simulink model "psk_rc_model"  (Simulink 8.7)
settings: Solver=FixedStepDiscrete  SolverMode=SingleTasking  StartTime=0.0  StopTime=1  FixedStep=1/100000  RelTol=1e-3  AbsTol=1e-6
undefined symbols (not defined in the file or in its folder): gcbh, rcfiltgaincompat
libraries: commfilt2 x1, dspsrcs4 x1
settings Model: Creator=amoura  LastModifiedBy=Artur Moura
settings DataIOCC: LimitDataPoints=off  SignalLoggingSaveFormat=ModelDataLogs
settings OptimizationCC: BlockReduction=off  BooleanDataType=off  ExpressionDepthLimit=2147483647  InitFltsAndDblsToZero=on
settings DebuggingCC: SaveWithParameterizedLinksMsg=none  SignalResolutionControl=TryResolveAllWithWarning  MultiTaskDSMMsg=warning  MultiTaskCondExecSysMsg=none  FcnCallInpInsideContextMsg=UseLocalSettings  StateNameClashWarn=warning
settings HardwareCC: TargetUnknown=on
settings RTWCC: TemplateMakefile=grt_unix.tmf
settings GRTTargetCC: TargetFcnLib=ansi_tfl_tmw.mat  ModelReferenceCompliant=off  CombineOutputUpdateFcns=off  MatFileLogging=off  GRTInterface=on

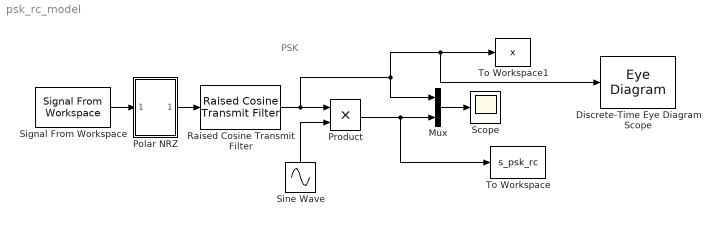
== system psk_rc_model ==
  note: PSK
  Discrete-Time Eye Diagram Scope : EyeDiagram  Tag=EyeDiagram
  Mux : Mux  Inputs=2
  Polar NRZ : Subsystem  mask(Polar NRZ){}
      mask help:
      | This block encodes a unipolar NRZ signal into the polar NRZ line code
      |
      | The output values are +1 for a nonzero input and -1 for a zero one.
      mask Display: disp('Polar\nNRZ')
  Product : Product  SaturateOnIntegerOverflow=on  RndMeth=Zero  InputSameDT=on  OutDataTypeStr=Inherit: Same as first input
  Raised Cosine Transmit Filter : commfilt2/Raised Cosine Transmit Filter  filtType=Normal  R=.3  filtSpan=2*(4)  N=100  filterGain=rcfiltgaincompat(gcbh)  InputProcessing=Columns as channels (frame based)  RateOptions=Allow multirate processing  framing=Mute  checkCoeff=off  variableName=rcTxFilt  checkGain=Normalized  sampMode=Mute  saveAsFlag=0  currentFiltSpan=2*(4)  D=4  launchFVT=off  roundingMode=Floor  overflowMode=off  coeffDataTypeStr=Inherit: Same word length as input  coeffMin=[]  coeffMax=[]  coeffLastDataTypeStr=Inherit: Same word length as input  outputDataTypeStr=Inherit: Same as accumulator  outputMin=[]  outputMax=[]  outputLastDataTypeStr=Inherit: Same as accumulator
  Scope : Scope
  Signal From Workspace : dspsrcs4/Signal From Workspace  X=randi([0 1],10000,1)  Ts=1/1000  nsamps=1  OutputAfterFinalValue=Cyclic repetition  ignoreOrWarnInputAndFrameLengths=off  OutputFrames=on
  Sine Wave : Sin  Frequency=2*pi*10000  SampleTime=0
  To Workspace : ToWorkspace  VariableName=s_psk_rc  SampleTime=1/100000
  To Workspace1 : ToWorkspace  VariableName=x  SampleTime=1/100000
  wires:
  Signal From Workspace/1 -> Polar NRZ/1(In1)
  Sine Wave/1 -> Product/2
  Product/1 -> To Workspace/1, Mux/2
  Polar NRZ/1(Out1) -> Raised Cosine Transmit Filter/1
  Raised Cosine Transmit Filter/1 -> Product/1, To Workspace1/1, Discrete-Time Eye Diagram Scope/1, Mux/1
  Mux/1 -> Scope/1

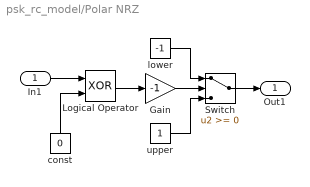
== system psk_rc_model/Polar NRZ ==
  In1 : Inport
  Gain : Gain  Gain=-1  SaturateOnIntegerOverflow=on  OutDataTypeStr=Inherit: Same as input  ParamDataTypeStr=Inherit: Same as input
  Logical Operator : Logic  Operator=XOR
  Switch : Switch  SaturateOnIntegerOverflow=on  InputSameDT=on
  const : Constant  Value=0
  lower : Constant  Value=-1
  upper : Constant
  Out1 : Outport  InitialOutput=0
  wires:
  const/1 -> Logical Operator/2
  Logical Operator/1 -> Gain/1
  Switch/1 -> Out1/1
  Gain/1 -> Switch/2
  upper/1 -> Switch/3
  lower/1 -> Switch/1
  In1/1 -> Logical Operator/1
